simulink model "testbed_R2019b"  (R2019b)
settings: Solver=VariableStepAuto  StartTime=0.0  StopTime=10.0  RelTol=1e-3
undefined symbols (not defined in the file or in its folder): ParAltimeter, ParCamera, ParRadio
settings Model: Creator=spectral000az  LastModifiedBy=spectral000az

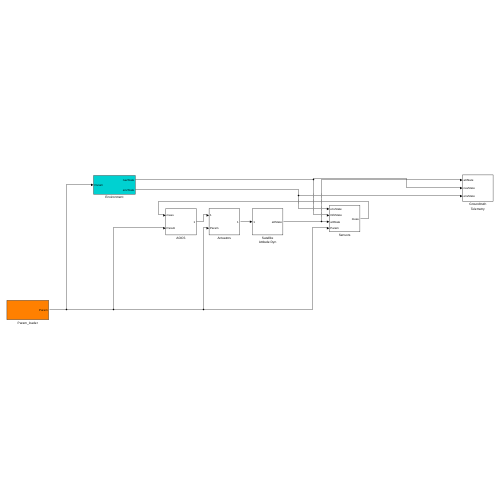
[thumbnail: Simulink's stored preview of the top-level diagram]
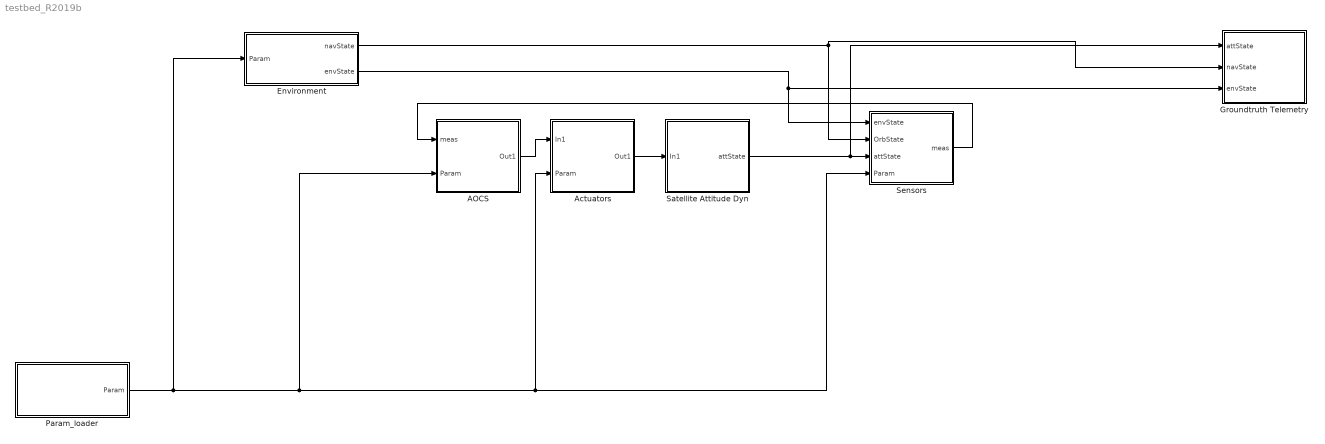
== system testbed_R2019b ==
  AOCS : Subsystem
  Actuators : Subsystem
  Environment : Subsystem
  Groundtruth Telemetry : Subsystem
  Param_loader : Subsystem
  Satellite Attitude Dyn : Subsystem
  Sensors : Subsystem
  wires:
  Actuators/1(Out1) -> Satellite Attitude Dyn/1(In1)
  AOCS/1(Out1) -> Actuators/1(In1)
  Environment/2(envState) -> Groundtruth Telemetry/3(envState), Sensors/1(envState)
  Environment/1(navState) -> Sensors/2(OrbState), Groundtruth Telemetry/2(navState)
  Param_loader/1(Param) -> Environment/1(Param), AOCS/2(Param), Actuators/2(Param), Sensors/4(Param)
  Satellite Attitude Dyn/1(attState) -> Groundtruth Telemetry/1(attState), Sensors/3(attState)
  Sensors/1(meas) -> AOCS/1(meas)

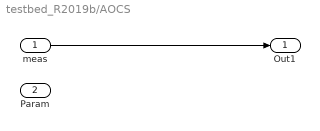
== system testbed_R2019b/AOCS ==
  meas : Inport
  Param : Inport  Port=2
  Out1 : Outport
  wires:
  meas/1 -> Out1/1

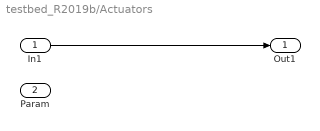
== system testbed_R2019b/Actuators ==
  In1 : Inport
  Param : Inport  Port=2
  Out1 : Outport
  wires:
  In1/1 -> Out1/1

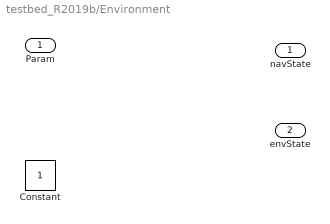
== system testbed_R2019b/Environment ==
  Param : Inport
  Constant : Constant
  navState : Outport
  envState : Outport  Port=2

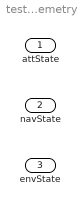
== system testbed_R2019b/Groundtruth Telemetry ==
  attState : Inport
  navState : Inport  Port=2
  envState : Inport  Port=3

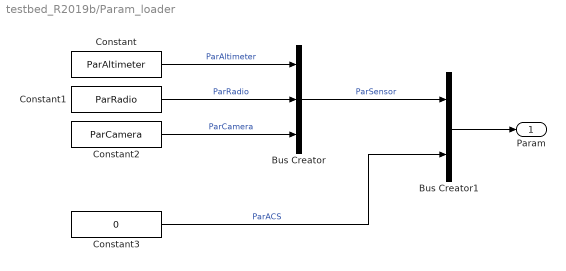
== system testbed_R2019b/Param_loader ==
  Bus Creator : BusCreator  Inputs=3
  Bus Creator1 : BusCreator  Inputs=2
  Constant : Constant  Value=ParAltimeter
  Constant1 : Constant  Value=ParRadio
  Constant2 : Constant  Value=ParCamera
  Constant3 : Constant  Value=0
  Param : Outport
  wires:
  Constant/1 -> Bus Creator/1  "ParAltimeter"
  Constant1/1 -> Bus Creator/2  "ParRadio"
  Constant2/1 -> Bus Creator/3  "ParCamera"
  Bus Creator/1 -> Bus Creator1/1  "ParSensor"
  Bus Creator1/1 -> Param/1
  Constant3/1 -> Bus Creator1/2  "ParACS"

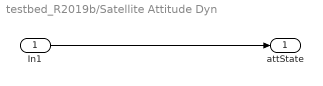
== system testbed_R2019b/Satellite Attitude Dyn ==
  In1 : Inport
  attState : Outport
  wires:
  In1/1 -> attState/1

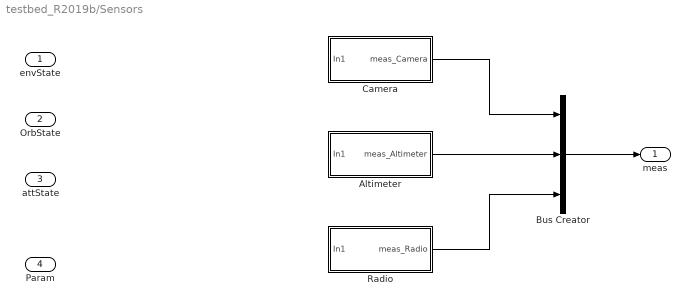
== system testbed_R2019b/Sensors ==
  envState : Inport
  OrbState : Inport  Port=2
  attState : Inport  Port=3
  Param : Inport  Port=4
  Altimeter : Subsystem
  Bus Creator : BusCreator  Inputs=3
  Camera : Subsystem
  Radio : Subsystem
  meas : Outport
  wires:
  Altimeter/1(meas_Altimeter) -> Bus Creator/2
  Camera/1(meas_Camera) -> Bus Creator/1
  Radio/1(meas_Radio) -> Bus Creator/3
  Bus Creator/1 -> meas/1

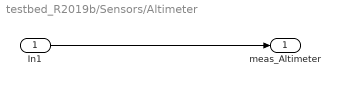
== system testbed_R2019b/Sensors/Altimeter ==
  In1 : Inport
  meas_Altimeter : Outport
  wires:
  In1/1 -> meas_Altimeter/1

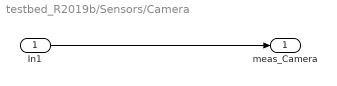
== system testbed_R2019b/Sensors/Camera ==
  In1 : Inport
  meas_Camera : Outport
  wires:
  In1/1 -> meas_Camera/1

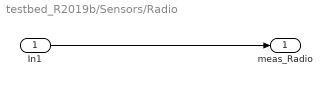
== system testbed_R2019b/Sensors/Radio ==
  In1 : Inport
  meas_Radio : Outport
  wires:
  In1/1 -> meas_Radio/1
